simulink model "Sensorik_Rob_Som25_03"  (R2024b)
settings: Solver=VariableStepAuto  StartTime=0.0  StopTime=1e-2  RelTol=1e-3
values from neighbouring files (symbols this model uses):
  C = 1e-6    (= 1e-06)    [Init_Sensorik.m]    (also in Sensorik_Rob_Som25_System.m)
  R = 1e3    (= 1000)    [Init_Sensorik.m]    (also in Sensorik_Rob_Som25_System.m)
libraries: fl_lib x6, nesl_utility x2
settings Model: Creator=turnwald  LastModifiedBy=turnwald

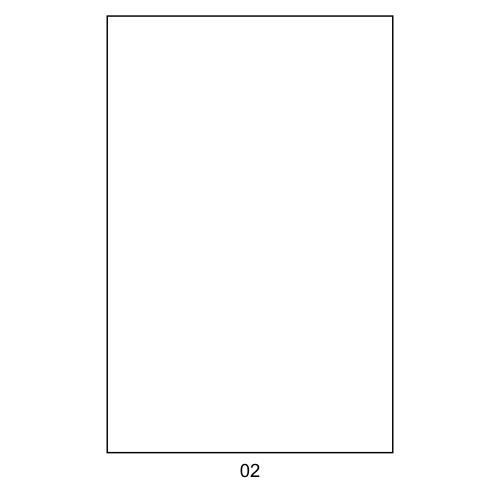
[thumbnail: Simulink's stored preview of the top-level diagram]
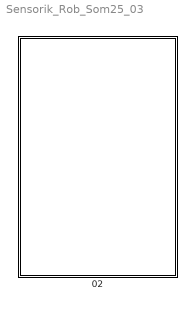
== system Sensorik_Rob_Som25_03 ==
  02 : Subsystem

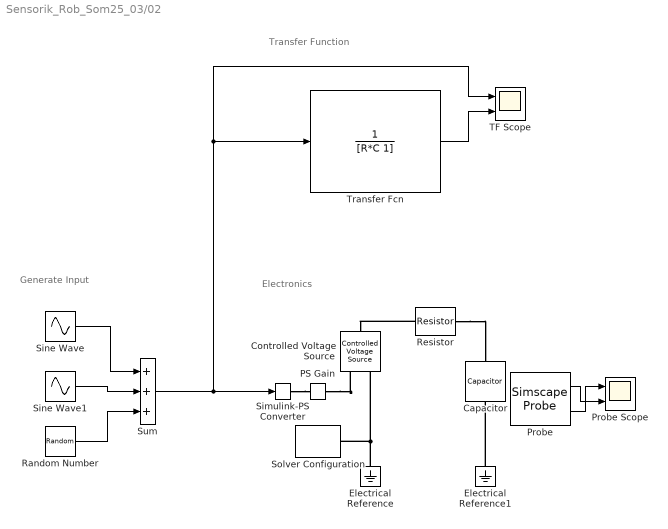
== system Sensorik_Rob_Som25_03/02 ==
  note: Generate Input
  note: Transfer Function
  note: Electronics
  Capacitor : fl_lib/Electrical/Electrical Elements/Capacitor  c=C F  r=0 Ohm  g=0 1/Ohm  i_specify=off  i_priority=None  i=0 A  i_nominal_specify=off  i_nominal_value=1  i_nominal_unit=A  v_specify=off  v_priority=None  v=0 V  v_nominal_specify=off  v_nominal_value=1  v_nominal_unit=V  vc_specify=off  vc_priority=High  vc=0 V  vc_nominal_specify=off  vc_nominal_value=1  vc_nominal_unit=V
  Controlled Voltage Source : fl_lib/Electrical/Electrical Sources/Controlled Voltage Source
  Electrical Reference : fl_lib/Electrical/Electrical Elements/Electrical Reference
  Electrical Reference1 : fl_lib/Electrical/Electrical Elements/Electrical Reference
  PS Gain : fl_lib/Physical Signals/Functions/PS Gain  gain=1
  Probe : SimscapeProbe  BoundBlock=79  Variables="{\"n.v\":{\"Unit\":\"V\",\"PortLabel\":\"n.v\",\"Probing\":\"ON\"},\"p.v\":{\"Unit\":\"V\",\"PortLabel\":\"p.v\",\"Probing\":\"ON\"}}"
  Probe Scope : Scope  NumInputPorts=2
  Random Number : RandomNumber  Variance=1e-2  SampleTime=1e-6
  Resistor : fl_lib/Electrical/Electrical Elements/Resistor  R=R Ohm  i_specify=off  i_priority=None  i=0 A  i_nominal_specify=off  i_nominal_value=1  i_nominal_unit=A  v_specify=off  v_priority=None  v=0 V  v_nominal_specify=off  v_nominal_value=1  v_nominal_unit=V
  Simulink-PS Converter : nesl_utility/Simulink-PS Converter  PhysicalDomain=network_engine_domain  SubClassName=ps_input  LeftPortType=input  RightPortType=output  PseudoPeriodic=off  Frequencies=[]  NoiseDistribution=none  NoiseParameters=[]  Unit=1  AffineConversion=off  FilteringAndDerivatives=provide  SimscapeFilterOrder=1  InputFilterTimeConstant=0.001  UdotUserProvided=0
  Sine Wave : Sin  Amplitude=5  Frequency=2*pi*100  SampleTime=0
  Sine Wave1 : Sin  Frequency=2*pi*2000  SampleTime=0
  Solver Configuration : nesl_utility/Solver Configuration  PhysicalDomain=network_engine_domain  SubClassName=solver  LeftPortType=input  RightPortType=generic  Tones=[]  Harmonics=[]  SimulateNoise=off  Profile=off  UseLocalSampling=off  EnableSwitchedLinearOptims=on  FrequencyDomain=off  UseCCode=off  RelTol=0.001  AbsTol=0.001  MinStep=1e-09  ToWorkspace=off  RevertToSquareIcSolve=off  NumHomotopyIterations=100  PhasorMode=off  PhasorModeNumHarmonics=1  ConsistencySolver=NEWTON_XTOL_AFTER_FTOL  IndexReductionMethod=DerivativeReplacement  DoDC=off  ResidualTolerance=1e-09  ConsistencyTolSource=GLOBAL  ConsistencyAbsTol=0.001  ConsistencyRelTol=0.001  ConsistencyTolFactor=0.001  UseLocalSolver=off  LocalSolverChoice=NE_BACKWARD_EULER_ADVANCER  ResolveIndetEquations=on  FunctionEvalNumThread=1  LocalSolverSampleTime=0.001  DoFixedCost=off  MaxNonlinIter=3  MaxModeIter=2  ComputeImpulses=off  ImpulseIterations=2  LinearAlgebra=auto  LinearAlgebraNumThread=0  EquationFormulation=NE_TIME_EF  DelaysMemoryBudget=1024  AutomaticFiltering=on  FilteringTimeConstant=0.001  PartitionStorageMethod=AS_NEEDED  PartitionMemoryBudget=1024  PartitionMethod=ROBUST  MultibodyUseLocalSolver=off  MultibodyLocalSolverChoice=ODE1  MultibodyLocalSolverSampleTime=0.001
  Sum : Sum  Inputs=+++
  TF Scope : Scope  NumInputPorts=2
  Transfer Fcn : TransferFcn  Denominator=[R*C 1]
  wires:
  Probe/2 -> Probe Scope/1
  Probe/1 -> Probe Scope/2
  Sum/1 -> TF Scope/1, Transfer Fcn/1, Simulink-PS Converter/1
  Sine Wave/1 -> Sum/1
  Sine Wave1/1 -> Sum/2
  Random Number/1 -> Sum/3
  Transfer Fcn/1 -> TF Scope/2
  connections:
  Resistor/RConn1 -- Capacitor/LConn1
  Electrical Reference1/LConn1 -- Capacitor/RConn1
  Electrical Reference/LConn1 -- Controlled Voltage Source/RConn2 -- Solver Configuration/RConn1
  Resistor/LConn1 -- Controlled Voltage Source/LConn1
  PS Gain/RConn1 -- Controlled Voltage Source/RConn1
  Simulink-PS Converter/RConn1 -- PS Gain/LConn1
